simulink model "SegwayV4_Combined"  (R2021a)
settings: Solver=ode45  StartTime=0.0  StopTime=5  RelTol=1e-3
values from neighbouring files (symbols this model uses):
  B = [0 ; B2 ; 0 ; B4;]    [Segway_modelV4.m]    (also in Segway_modelV6.m)
  C = [1 0 0 0 ... (first row only)    [Segway_modelV4.m]    (also in Segway_modelV6.m)
  r = 1.6    [Segway_modelV4.m]    (also in Segway_modelV6.m)
  tf_turn = tf(Km,[r*Iw,Km*Ke,0])    [Segway_modelV4.m]    (also in Segway_modelV6.m)
  Theta_req = arr(i)    [Segway_modelV6.m]
  X0 = [0 ;0 ;0 ;0;]    [Segway_modelV4.m]    (also in Segway_modelV6.m)
  X_req = 10    [Segway_modelV6.m]
undefined symbols (not defined in the file or in its folder): K
libraries: pid_lib x1
settings Model: Creator=Akshit  LastModifiedBy=mluser
settings SolverCC: AlgebraicLoopSolver=TrustRegion
settings DataIOCC: ReturnWorkspaceOutputs=off
settings DebuggingCC: SFMachineParentedDataDiag=warning

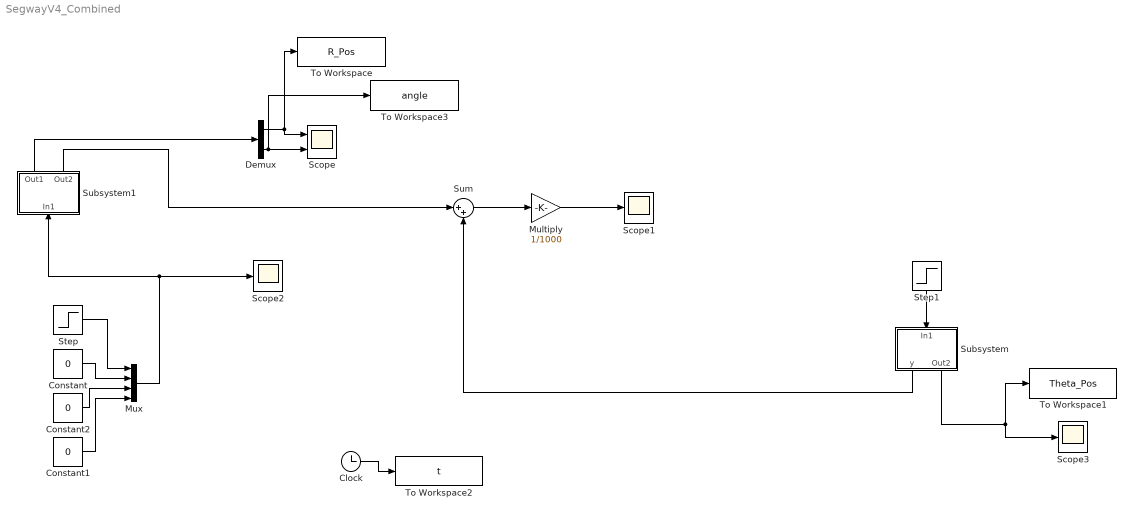
== system SegwayV4_Combined ==
  Clock : Clock
  Constant : Constant  Value=0
  Constant1 : Constant  Value=0
  Constant2 : Constant  Value=0
  Demux : Demux  Outputs=2
  Multiply : Gain  Gain=1/1000
  Mux : Mux
  Scope : Scope  NumInputPorts=2
  Scope1 : Scope
  Scope2 : Scope
  Scope3 : Scope
  Step : Step  Time=2  After=X_req  SampleTime=0
  Step1 : Step  Time=0  After=Theta_req  SampleTime=0
  Subsystem : Subsystem
  Subsystem1 : Subsystem
  Sum : Sum  Inputs=|++
  To Workspace : ToWorkspace  VariableName=R_Pos  SaveFormat=Timeseries  SampleTime=-1
  To Workspace1 : ToWorkspace  VariableName=Theta_Pos  SaveFormat=Timeseries  SampleTime=-1
  To Workspace2 : ToWorkspace  VariableName=t  SaveFormat=Timeseries  SampleTime=-1
  To Workspace3 : ToWorkspace  VariableName=angle  SaveFormat=Timeseries  SampleTime=-1
  wires:
  Step/1 -> Mux/1
  Constant/1 -> Mux/2
  Constant1/1 -> Mux/4
  Constant2/1 -> Mux/3
  Demux/1 -> To Workspace/1, Scope/1
  Subsystem/2(Out2) -> Scope3/1, To Workspace1/1
  Step1/1 -> Subsystem/1(In1)
  Subsystem1/1(Out1) -> Demux/1
  Subsystem1/2(Out2) -> Sum/1
  Subsystem/1(y) -> Sum/2
  Mux/1 -> Subsystem1/1(In1), Scope2/1
  Clock/1 -> To Workspace2/1
  Multiply/1 -> Scope1/1
  Sum/1 -> Multiply/1
  Demux/2 -> To Workspace3/1, Scope/2

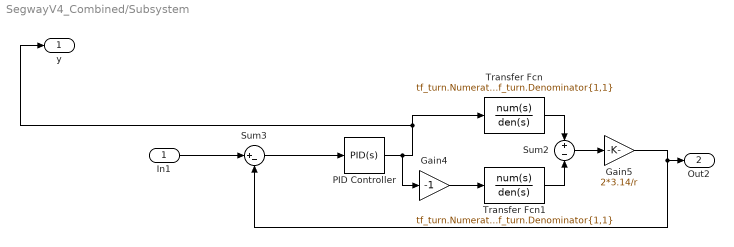
== system SegwayV4_Combined/Subsystem ==
  In1 : Inport
  Gain4 : Gain  Gain=-1
  Gain5 : Gain  Gain=2*3.14/r
  PID Controller : pid_lib/PID Controller  Controller=PID  Form=Parallel  TimeDomain=Continuous-time  UseExternalTs=off  SampleTime=-1  IntegratorMethod=Forward Euler  FilterMethod=Forward Euler  ControllerParametersSource=internal  P=0.56326  I=5.9454  D=0.32903  UseFilter=on  N=100  TunerSelectOption=Transfer Function Based (PID Tuner App)  InitialConditionSource=internal  InitialConditionForIntegrator=0  InitialConditionForFilter=0  DifferentiatorICPrevScaledInput=0  ExternalReset=none  TrackingMode=off  Kt=1  LimitOutput=off  SatLimitsSource=internal  UpperSaturationLimit=inf  LowerSaturationLimit=-inf  LinearizeAsGain=on  AntiWindupMode=none  Kb=1  POutMin=[]  POutMax=[]  IOutMin=[]  IOutMax=[]  DOutMin=[]  DOutMax=[]  NOutMin=[]  NOutMax=[]  SumOutMin=[]  SumOutMax=[]  SaturationOutMin=[]  SaturationOutMax=[]  PParamMin=[]  PParamMax=[]  IParamMin=[]  IParamMax=[]  DParamMin=[]  DParamMax=[]  NParamMin=[]  NParamMax=[]  KbParamMin=[]  KbParamMax=[]  KtParamMin=[]  KtParamMax=[]  KbOutMin=[]  KbOutMax=[]  KtOutMin=[]  KtOutMax=[]  IntegratorOutMin=[]  IntegratorOutMax=[]  FilterOutMin=[]  FilterOutMax=[]  SumI1OutMin=[]  SumI1OutMax=[]  SumI2OutMin=[]  SumI2OutMax=[]  SumI3OutMin=[]  SumI3OutMax=[]  SumI4OutMin=[]  SumI4OutMax=[]  SumDOutMin=[]  SumDOutMax=[]  DifferentiatorOutMin=[]  DifferentiatorOutMax=[]  FilterDiffOutCoefMin=[]  FilterDiffOutCoefMax=[]  ReciprocalOutMin=[]  ReciprocalOutMax=[]  SumDenOutMin=[]  SumDenOutMax=[]  SumNumOutMin=[]  SumNumOutMax=[]  DivideOutMin=[]  DivideOutMax=[]  UdiffTsProdOutMin=[]  UdiffTsProdOutMax=[]  NTsProdOutMin=[]  NTsProdOutMax=[]  UintegralTsProdOutMin=[]  UintegralTsProdOutMax=[]  UngainTsProdOutMin=[]  UngainTsProdOutMax=[]  IntegratorContinuousStateAttributes=''  IntegratorStateMustResolveToSignalObject=off  IntegratorRTWStateStorageClass=Auto  FilterContinuousStateAttributes=''  FilterStateMustResolveToSignalObject=off  FilterRTWStateStorageClass=Auto  ParallelPVariant=InternalParameters  IdealPVariant=Disabled  IVariant=InternalParameters  DVariant=InternalParameters  IntegratorVariant=Continuous  SatVariant=Disabled  AWVariant=Passthrough  PCopyVariant=Disabled  TRVariant=Disabled  FdbkBlocksVariant=Forward  IdealPFdbkVariant=Disabled  SatFdbkVariant=Disabled  DerivativeFilterVariant=ContFilter  NVariant=InternalParameters  NCopyVariant=Disabled  FilterICVariant=InternalICsFilter  IntegratorICVariant=InternalICs  ExternalResetVariant=Disabled  TRSumVariant=Passthrough  SumFdbkVariant=Disabled  SumVariant=Sum_PID  TsampFilterVariant=InternalTs  TsampNgainVariant=Passthrough  TsampIntegralVariant=Passthrough  ExternalSaturationOutDataTypeStr=Inherit: Same as second input
  Sum2 : Sum  Inputs=+-
  Sum3 : Sum  Inputs=|+-
  Transfer Fcn : TransferFcn  Numerator=tf_turn.Numerator{1,1}  Denominator=tf_turn.Denominator{1,1}
  Transfer Fcn1 : TransferFcn  Numerator=tf_turn.Numerator{1,1}  Denominator=tf_turn.Denominator{1,1}
  y : Outport
  Out2 : Outport  Port=2
  wires:
  Sum3/1 -> PID Controller/1
  PID Controller/1 -> y/1, Transfer Fcn/1, Gain4/1
  In1/1 -> Sum3/1
  Gain4/1 -> Transfer Fcn1/1
  Sum2/1 -> Gain5/1
  Transfer Fcn/1 -> Sum2/1
  Gain5/1 -> Out2/1, Sum3/2
  Transfer Fcn1/1 -> Sum2/2

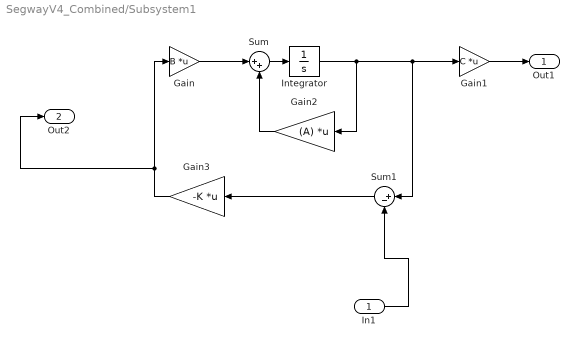
== system SegwayV4_Combined/Subsystem1 ==
  In1 : Inport
  Gain : Gain  Gain=B  Multiplication=Matrix(K*u)
  Gain1 : Gain  Gain=C  Multiplication=Matrix(K*u)
  Gain2 : Gain  Gain=(A)  Multiplication=Matrix(K*u)
  Gain3 : Gain  Gain=-K  Multiplication=Matrix(K*u)
  Integrator : Integrator  InitialCondition=X0
  Sum : Sum  Inputs=|++
  Sum1 : Sum  Inputs=|+-
  Out1 : Outport
  Out2 : Outport  Port=2
  wires:
  Sum1/1 -> Gain3/1
  Integrator/1 -> Gain2/1, Sum1/1, Gain1/1
  Gain1/1 -> Out1/1
  Gain3/1 -> Out2/1, Gain/1
  Gain2/1 -> Sum/2
  Sum/1 -> Integrator/1
  Gain/1 -> Sum/1
  In1/1 -> Sum1/2
